simulink model "EventBasedTransmition"  (R2024a)
settings: Solver=VariableStepDiscrete  StartTime=0.0  StopTime=10  RelTol=1e-3
undefined symbols (not defined in the file): canChannel
libraries: canlib x2, canmsglib x2, simulink x1
settings Model: Creator=The MathWorks, Inc.  LastModifiedBy=prat
settings SolverCC: AlgebraicLoopSolver=TrustRegion  MaxZcPerStep=1
settings DebuggingCC: UnconnectedInputMsg=warning  UnconnectedOutputMsg=warning  UnconnectedLineMsg=warning
settings ModelReferenceCC: EnableRefExpFcnMdlSchedulingChecks=on
settings RTWCC: GPUComputeCapability=3.5  DLArmComputeVersion=19.05

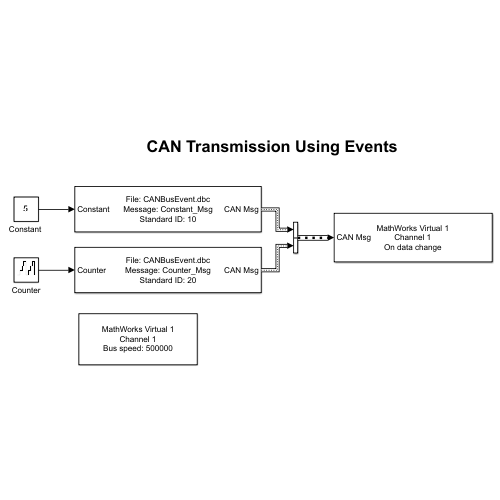
[thumbnail: Simulink's stored preview of the top-level diagram]
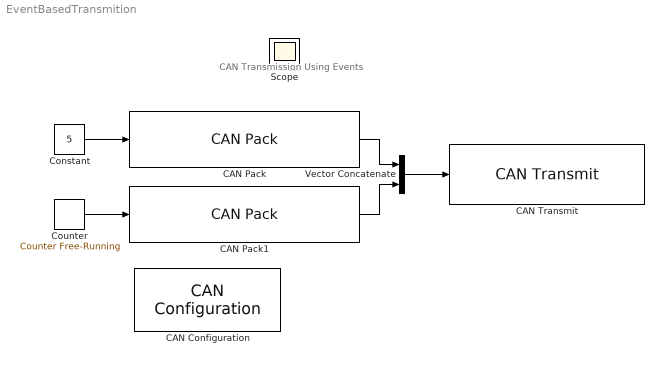
== system EventBasedTransmition ==
  note: CAN Transmission Using Events
  CAN Configuration : canlib/CAN Configuration  BlockHandle=164.0001  Device=MathWorks Virtual 1 (Channel 1)  DeviceMenu=MathWorks Virtual 1 (Channel 1)  ObjConstructor=canChannel('MathWorks', 'Virtual 1', 1)  BusSpeed=500000  EnableBitParameters=off  AckMode=Normal
  CAN Pack : canmsglib/CAN Pack  CANdbFile=CANBusEvent.dbc  MsgList=Constant_Msg  MsgName=Constant_Msg  MsgIDType=Standard (11-bit identifier)  MsgIdentifier=10  MsgLength=4  Remote=off  ApplyMinMax=off  BusOutput=on  SignalInfo={'Constant','0','32','LE','unsigned','Standard','0','1','0','0','4294967295'}
      settings: DataFormat=CANdb specified signals
  CAN Pack1 : canmsglib/CAN Pack  CANdbFile=CANBusEvent.dbc  MsgList=Counter_Msg  MsgName=Counter_Msg  MsgIDType=Standard (11-bit identifier)  MsgIdentifier=20  MsgLength=4  Remote=off  ApplyMinMax=off  BusOutput=on  SignalInfo={'Counter','0','32','LE','unsigned','Standard','0','1','0','0','4294967295'}
      settings: DataFormat=CANdb specified signals
  CAN Transmit : canlib/CAN Transmit  BlockHandle=171.0001  Device=MathWorks Virtual 1 (Channel 1)  DeviceMenu=MathWorks Virtual 1 (Channel 1)  ObjConstructor=canChannel('MathWorks', 'Virtual 1', 1)  EnableEventTransmit=on  EnablePeriodicTransmit=off  MessagePeriod=0.100
  "Constant " : Constant  Value=5  OutDataTypeStr=uint8
  Counter : simulink/Sources/Counter Free-Running  NumBits=32  tsamp=1
  Vector Concatenate : Concatenate
  Scope : Scope
  wires:
  CAN Pack/1 -> Vector Concatenate/1
  Counter/1 -> CAN Pack1/1
  CAN Pack1/1 -> Vector Concatenate/2
  Vector Concatenate/1 -> CAN Transmit/1
  "Constant "/1 -> CAN Pack/1
